simulink model "MPS_device_passive"  (R2018b)
settings: Solver=ode4  StartTime=0  StopTime=700  FixedStep=0.02  MaxStep=0.02  RelTol=1e-3  EnableMultiTasking=on
InitFcn:
  | %SSModel_calc
undefined symbols (not defined in the file): body, CentralPTOPreload, constraint, L, ML1Preload, ML2Preload, ML3Preload, ML4Preload, ML5Preload, ML6Preload, ML7Preload, ML8Preload, mrelative, pto, PTOrotation, SidePTO1Preload, SidePTO2Preload, SidePTO3Preload, SidePTO4Preload, simu, waves, X, Y, Z
libraries: nesl_utility x580, sm_lib x317, vrlib x72, WECSim_Lib x36
(part 24 of 27)

== system MPS_device_passive/PTO P2F2/VisuP2F3/Hydrodynamic Body/Morrison Element and ViscousDampingForceCalculation/Morrison Element Variant Subsystem/Morrison Element On/No Wave Morison Force/MorrisonElements/Rotation1 ==
  rot1 : Inport
  rot2 : Inport  Port=2
  rot3 : Inport  Port=3
  2 : Product
  3 : Product  Inputs=3
  7 : Product
  8 : Product  Inputs=3
  Combine : Concatenate  NumInputs=3  Mode=Multidimensional array  ConcatenateDimension=2
  Trigonometric Function{,1..2,6,9,11} (6 alike) : Trigonometry  Operator=cos
  Trigonometric Function{3..5,7..8,10} (6 alike) : Trigonometry
  rot11 : Product
  rot12 : Sum
  rot13 : Sum  Inputs=+-
  rot[1,1-3] : Outport
  wires:
  rot13/1 -> Combine/3
  8/1 -> rot13/2
  7/1 -> rot13/1
  Trigonometric Function11/1 -> 8/3
  Trigonometric Function10/1 -> 8/2
  Trigonometric Function9/1 -> 8/1
  Trigonometric Function8/1 -> 7/2
  Trigonometric Function7/1 -> 7/1
  rot1/1 -> Trigonometric Function7/1, Trigonometric Function9/1, Trigonometric Function4/1, Trigonometric Function2/1
  rot3/1 -> Trigonometric Function8/1, Trigonometric Function11/1, Trigonometric Function6/1, Trigonometric Function3/1, Trigonometric Function1/1
  rot2/1 -> Trigonometric Function10/1, Trigonometric Function5/1, Trigonometric Function/1
  Combine/1 -> rot[1,1-3]/1
  rot12/1 -> Combine/2
  3/1 -> rot12/2
  2/1 -> rot12/1
  Trigonometric Function6/1 -> 3/3
  Trigonometric Function5/1 -> 3/2
  Trigonometric Function4/1 -> 3/1
  Trigonometric Function3/1 -> 2/2
  Trigonometric Function2/1 -> 2/1
  rot11/1 -> Combine/1
  Trigonometric Function1/1 -> rot11/2
  Trigonometric Function/1 -> rot11/1

== system MPS_device_passive/PTO P2F2/VisuP2F3/Hydrodynamic Body/Morrison Element and ViscousDampingForceCalculation/Morrison Element Variant Subsystem/Morrison Element On/No Wave Morison Force/MorrisonElements/Rotation2 ==
  rot1 : Inport
  rot2 : Inport  Port=2
  rot3 : Inport  Port=3
  2 : Product
  3 : Product  Inputs=3
  7 : Product
  8 : Product  Inputs=3
  Combine : Concatenate  NumInputs=3  Mode=Multidimensional array  ConcatenateDimension=2
  Gain : Gain  Gain=-1
  Trigonometric Function{,2..3,8..9} (5 alike) : Trigonometry  Operator=cos
  Trigonometric Function{1,4..7,10..11} (7 alike) : Trigonometry
  rot11 : Product
  rot12 : Sum  Inputs=+-
  rot13 : Sum
  rot[2,1-3] : Outport
  wires:
  Gain/1 -> rot11/1
  rot13/1 -> Combine/3
  8/1 -> rot13/2
  7/1 -> rot13/1
  Trigonometric Function11/1 -> 8/3
  Trigonometric Function10/1 -> 8/2
  Trigonometric Function9/1 -> 8/1
  Trigonometric Function8/1 -> 7/2
  Trigonometric Function7/1 -> 7/1
  rot1/1 -> Trigonometric Function7/1, Trigonometric Function9/1, Trigonometric Function4/1, Trigonometric Function2/1
  rot3/1 -> Trigonometric Function8/1, Trigonometric Function11/1, Trigonometric Function6/1, Trigonometric Function3/1, Trigonometric Function1/1
  rot2/1 -> Trigonometric Function10/1, Trigonometric Function5/1, Trigonometric Function/1
  Combine/1 -> rot[2,1-3]/1
  rot12/1 -> Combine/2
  3/1 -> rot12/2
  2/1 -> rot12/1
  Trigonometric Function6/1 -> 3/3
  Trigonometric Function5/1 -> 3/2
  Trigonometric Function4/1 -> 3/1
  Trigonometric Function3/1 -> 2/2
  Trigonometric Function2/1 -> 2/1
  rot11/1 -> Combine/1
  Trigonometric Function1/1 -> rot11/2
  Trigonometric Function/1 -> Gain/1

== system MPS_device_passive/PTO P2F2/VisuP2F3/Hydrodynamic Body/Morrison Element and ViscousDampingForceCalculation/Morrison Element Variant Subsystem/Morrison Element On/No Wave Morison Force/MorrisonElements/Rotation3 ==
  rot1 : Inport
  rot2 : Inport  Port=2
  2 : Product
  7 : Product
  Combine : Concatenate  NumInputs=3  Mode=Multidimensional array  ConcatenateDimension=2
  Gain1 : Gain  Gain=-1
  TrigFun1 : Trigonometry
  TrigFun2 : Trigonometry
  TrigFun3 : Trigonometry  Operator=cos
  TrigFun4 : Trigonometry  Operator=cos
  TrigFun5 : Trigonometry  Operator=cos
  rot[3,1-3] : Outport
  wires:
  Gain1/1 -> 2/1
  TrigFun2/1 -> Gain1/1
  7/1 -> Combine/3
  rot1/1 -> TrigFun4/1, TrigFun2/1
  TrigFun5/1 -> 7/2
  TrigFun4/1 -> 7/1
  rot2/1 -> TrigFun1/1, TrigFun3/1, TrigFun5/1
  Combine/1 -> rot[3,1-3]/1
  2/1 -> Combine/2
  TrigFun3/1 -> 2/2
  TrigFun1/1 -> Combine/1

== system MPS_device_passive/PTO P2F2/VisuP2F3/Hydrodynamic Body/Morrison Element and ViscousDampingForceCalculation/Morrison Element Variant Subsystem/Morrison Element On/Regular Wave Morison Force/MorrisonElements/OrbitalVelocity ==
  Disp : Inport
  Time : Inport  Port=2
  MATLAB Function : MATLAB Function  TreatAsAtomicUnit=on
  WaveAmp : Constant  Value=waves.A(1,:)
  WaveFreq : Constant  Value=waves.w(1,:)
  WaveNumber : Constant  Value=waves.k(1,:)
  gravity : Constant  Value=simu.g  VectorParams1D=off
  phase : Constant  Value=0
  rampTime : Constant  Value=simu.rampT  VectorParams1D=off
  waterDepth : Constant  Value=waves.waterDepth  VectorParams1D=off
  waveDirection : Constant  Value=waves.waveDir  VectorParams1D=off
  u-V : Outport
  w-V : Outport  Port=2
  u-A : Outport  Port=3
  w-A : Outport  Port=4
  v-V : Outport  Port=5
  v-A : Outport  Port=6
  wires:
  MATLAB Function/5(ya) -> v-A/1
  MATLAB Function/1(u) -> u-V/1
  MATLAB Function/2(v) -> v-V/1
  MATLAB Function/6(za) -> w-A/1
  MATLAB Function/4(xa) -> u-A/1
  MATLAB Function/3(w) -> w-V/1
  rampTime/1 -> MATLAB Function/7(rampT)
  waveDirection/1 -> MATLAB Function/8(waveDir)
  waterDepth/1 -> MATLAB Function/9(waterDepth)
  gravity/1 -> MATLAB Function/10(g)
  Time/1 -> MATLAB Function/6(time)
  WaveAmp/1 -> MATLAB Function/4(waveAmp)
  WaveFreq/1 -> MATLAB Function/3(waveFreq)
  WaveNumber/1 -> MATLAB Function/2(waveNumber)
  phase/1 -> MATLAB Function/5(randPhase)
  Disp/1 -> MATLAB Function/1(disp)

== system MPS_device_passive/PTO P2F2/VisuP2F3/Hydrodynamic Body/Morrison Element and ViscousDampingForceCalculation/Morrison Element Variant Subsystem/Morrison Element On/Regular Wave Morison Force/MorrisonElements/Rotation1 ==
  rot1 : Inport
  rot2 : Inport  Port=2
  rot3 : Inport  Port=3
  2 : Product
  3 : Product  Inputs=3
  7 : Product
  8 : Product  Inputs=3
  Combine : Concatenate  NumInputs=3  Mode=Multidimensional array  ConcatenateDimension=2
  Trigonometric Function{,1..2,6,9,11} (6 alike) : Trigonometry  Operator=cos
  Trigonometric Function{3..5,7..8,10} (6 alike) : Trigonometry
  rot11 : Product
  rot12 : Sum
  rot13 : Sum  Inputs=+-
  rot[1,1-3] : Outport
  wires:
  rot13/1 -> Combine/3
  8/1 -> rot13/2
  7/1 -> rot13/1
  Trigonometric Function11/1 -> 8/3
  Trigonometric Function10/1 -> 8/2
  Trigonometric Function9/1 -> 8/1
  Trigonometric Function8/1 -> 7/2
  Trigonometric Function7/1 -> 7/1
  rot1/1 -> Trigonometric Function7/1, Trigonometric Function9/1, Trigonometric Function4/1, Trigonometric Function2/1
  rot3/1 -> Trigonometric Function8/1, Trigonometric Function11/1, Trigonometric Function6/1, Trigonometric Function3/1, Trigonometric Function1/1
  rot2/1 -> Trigonometric Function10/1, Trigonometric Function5/1, Trigonometric Function/1
  Combine/1 -> rot[1,1-3]/1
  rot12/1 -> Combine/2
  3/1 -> rot12/2
  2/1 -> rot12/1
  Trigonometric Function6/1 -> 3/3
  Trigonometric Function5/1 -> 3/2
  Trigonometric Function4/1 -> 3/1
  Trigonometric Function3/1 -> 2/2
  Trigonometric Function2/1 -> 2/1
  rot11/1 -> Combine/1
  Trigonometric Function1/1 -> rot11/2
  Trigonometric Function/1 -> rot11/1

== system MPS_device_passive/PTO P2F2/VisuP2F3/Hydrodynamic Body/Morrison Element and ViscousDampingForceCalculation/Morrison Element Variant Subsystem/Morrison Element On/Regular Wave Morison Force/MorrisonElements/Rotation2 ==
  rot1 : Inport
  rot2 : Inport  Port=2
  rot3 : Inport  Port=3
  2 : Product
  3 : Product  Inputs=3
  7 : Product
  8 : Product  Inputs=3
  Combine : Concatenate  NumInputs=3  Mode=Multidimensional array  ConcatenateDimension=2
  Gain : Gain  Gain=-1
  Trigonometric Function{,2..3,8..9} (5 alike) : Trigonometry  Operator=cos
  Trigonometric Function{1,4..7,10..11} (7 alike) : Trigonometry
  rot11 : Product
  rot12 : Sum  Inputs=+-
  rot13 : Sum
  rot[2,1-3] : Outport
  wires:
  Gain/1 -> rot11/1
  rot13/1 -> Combine/3
  8/1 -> rot13/2
  7/1 -> rot13/1
  Trigonometric Function11/1 -> 8/3
  Trigonometric Function10/1 -> 8/2
  Trigonometric Function9/1 -> 8/1
  Trigonometric Function8/1 -> 7/2
  Trigonometric Function7/1 -> 7/1
  rot1/1 -> Trigonometric Function7/1, Trigonometric Function9/1, Trigonometric Function4/1, Trigonometric Function2/1
  rot3/1 -> Trigonometric Function8/1, Trigonometric Function11/1, Trigonometric Function6/1, Trigonometric Function3/1, Trigonometric Function1/1
  rot2/1 -> Trigonometric Function10/1, Trigonometric Function5/1, Trigonometric Function/1
  Combine/1 -> rot[2,1-3]/1
  rot12/1 -> Combine/2
  3/1 -> rot12/2
  2/1 -> rot12/1
  Trigonometric Function6/1 -> 3/3
  Trigonometric Function5/1 -> 3/2
  Trigonometric Function4/1 -> 3/1
  Trigonometric Function3/1 -> 2/2
  Trigonometric Function2/1 -> 2/1
  rot11/1 -> Combine/1
  Trigonometric Function1/1 -> rot11/2
  Trigonometric Function/1 -> Gain/1

== system MPS_device_passive/PTO P2F2/VisuP2F3/Hydrodynamic Body/Morrison Element and ViscousDampingForceCalculation/Morrison Element Variant Subsystem/Morrison Element On/Regular Wave Morison Force/MorrisonElements/Rotation3 ==
  rot1 : Inport
  rot2 : Inport  Port=2
  2 : Product
  7 : Product
  Combine : Concatenate  NumInputs=3  Mode=Multidimensional array  ConcatenateDimension=2
  Gain1 : Gain  Gain=-1
  TrigFun1 : Trigonometry
  TrigFun2 : Trigonometry
  TrigFun3 : Trigonometry  Operator=cos
  TrigFun4 : Trigonometry  Operator=cos
  TrigFun5 : Trigonometry  Operator=cos
  rot[3,1-3] : Outport
  wires:
  Gain1/1 -> 2/1
  TrigFun2/1 -> Gain1/1
  7/1 -> Combine/3
  rot1/1 -> TrigFun4/1, TrigFun2/1
  TrigFun5/1 -> 7/2
  TrigFun4/1 -> 7/1
  rot2/1 -> TrigFun1/1, TrigFun3/1, TrigFun5/1
  Combine/1 -> rot[3,1-3]/1
  2/1 -> Combine/2
  TrigFun3/1 -> 2/2
  TrigFun1/1 -> Combine/1

== system MPS_device_passive/PTO P3F3/VisuP3F2/Hydrodynamic Body/Morrison Element and ViscousDampingForceCalculation/Morrison Element Variant Subsystem/Morrison Element On/Irregular Wave Morison Force/MorrisonElements/MorisonElementIrregular ==
  Disp : Inport
  waves.kirr : Inport  Port=2  Partition=on  PartitionDimension=1  PartitionWidth=1  PartitionOffset=0
  waves.w : Inport  Port=3  Partition=on  PartitionDimension=1  PartitionWidth=1  PartitionOffset=0
  waves.A : Inport  Port=4  Partition=on  PartitionDimension=1  PartitionWidth=1  PartitionOffset=0
  waves.RandPhase : Inport  Port=5  Partition=on  PartitionDimension=1  PartitionWidth=1  PartitionOffset=0
  Time : Inport  Port=6
  For Each : ForEach  DisableCoverage=on  IndexMode=One-based
  MATLAB Function : MATLAB Function  TreatAsAtomicUnit=on
  gravity : Constant  Value=simu.g  VectorParams1D=off
  rampTime : Constant  Value=simu.rampT  VectorParams1D=off
  waterDepth : Constant  Value=waves.waterDepth  VectorParams1D=off
  waveDirection : Constant  Value=waves.waveDir  VectorParams1D=off
  u-V : Outport  ConcatenationDimension=1
  w-V : Outport  Port=2  ConcatenationDimension=1
  x-A : Outport  Port=3  ConcatenationDimension=1
  w-A : Outport  Port=4  ConcatenationDimension=1
  v-V : Outport  Port=5  ConcatenationDimension=1
  y-A : Outport  Port=6  ConcatenationDimension=1
  wires:
  MATLAB Function/3(w) -> w-V/1
  MATLAB Function/4(xa) -> x-A/1
  MATLAB Function/6(za) -> w-A/1
  MATLAB Function/5(ya) -> y-A/1
  MATLAB Function/2(v) -> v-V/1
  Time/1 -> MATLAB Function/6(time)
  waves.kirr/1 -> MATLAB Function/2(waveNumber)
  MATLAB Function/1(u) -> u-V/1
  waves.RandPhase/1 -> MATLAB Function/5(randPhase)
  waves.A/1 -> MATLAB Function/4(waveAmp)
  waves.w/1 -> MATLAB Function/3(waveFreq)
  Disp/1 -> MATLAB Function/1(disp)
  rampTime/1 -> MATLAB Function/7(rampT)
  waveDirection/1 -> MATLAB Function/8(waveDir)
  waterDepth/1 -> MATLAB Function/9(waterDepth)
  gravity/1 -> MATLAB Function/10(g)

== system MPS_device_passive/PTO P3F3/VisuP3F2/Hydrodynamic Body/Morrison Element and ViscousDampingForceCalculation/Morrison Element Variant Subsystem/Morrison Element On/Irregular Wave Morison Force/MorrisonElements/Rotation1 ==
  rot1 : Inport
  rot2 : Inport  Port=2
  rot3 : Inport  Port=3
  2 : Product
  3 : Product  Inputs=3
  7 : Product
  8 : Product  Inputs=3
  Combine : Concatenate  NumInputs=3  Mode=Multidimensional array  ConcatenateDimension=2
  Trigonometric Function{,1..2,6,9,11} (6 alike) : Trigonometry  Operator=cos
  Trigonometric Function{3..5,7..8,10} (6 alike) : Trigonometry
  rot11 : Product
  rot12 : Sum
  rot13 : Sum  Inputs=+-
  rot[1,1-3] : Outport
  wires:
  rot13/1 -> Combine/3
  8/1 -> rot13/2
  7/1 -> rot13/1
  Trigonometric Function11/1 -> 8/3
  Trigonometric Function10/1 -> 8/2
  Trigonometric Function9/1 -> 8/1
  Trigonometric Function8/1 -> 7/2
  Trigonometric Function7/1 -> 7/1
  rot1/1 -> Trigonometric Function7/1, Trigonometric Function9/1, Trigonometric Function4/1, Trigonometric Function2/1
  rot3/1 -> Trigonometric Function8/1, Trigonometric Function11/1, Trigonometric Function6/1, Trigonometric Function3/1, Trigonometric Function1/1
  rot2/1 -> Trigonometric Function10/1, Trigonometric Function5/1, Trigonometric Function/1
  Combine/1 -> rot[1,1-3]/1
  rot12/1 -> Combine/2
  3/1 -> rot12/2
  2/1 -> rot12/1
  Trigonometric Function6/1 -> 3/3
  Trigonometric Function5/1 -> 3/2
  Trigonometric Function4/1 -> 3/1
  Trigonometric Function3/1 -> 2/2
  Trigonometric Function2/1 -> 2/1
  rot11/1 -> Combine/1
  Trigonometric Function1/1 -> rot11/2
  Trigonometric Function/1 -> rot11/1

== system MPS_device_passive/PTO P3F3/VisuP3F2/Hydrodynamic Body/Morrison Element and ViscousDampingForceCalculation/Morrison Element Variant Subsystem/Morrison Element On/Irregular Wave Morison Force/MorrisonElements/Rotation2 ==
  rot1 : Inport
  rot2 : Inport  Port=2
  rot3 : Inport  Port=3
  2 : Product
  3 : Product  Inputs=3
  7 : Product
  8 : Product  Inputs=3
  Combine : Concatenate  NumInputs=3  Mode=Multidimensional array  ConcatenateDimension=2
  Gain : Gain  Gain=-1
  Trigonometric Function{,2..3,8..9} (5 alike) : Trigonometry  Operator=cos
  Trigonometric Function{1,4..7,10..11} (7 alike) : Trigonometry
  rot11 : Product
  rot12 : Sum  Inputs=+-
  rot13 : Sum
  rot[2,1-3] : Outport
  wires:
  Gain/1 -> rot11/1
  rot13/1 -> Combine/3
  8/1 -> rot13/2
  7/1 -> rot13/1
  Trigonometric Function11/1 -> 8/3
  Trigonometric Function10/1 -> 8/2
  Trigonometric Function9/1 -> 8/1
  Trigonometric Function8/1 -> 7/2
  Trigonometric Function7/1 -> 7/1
  rot1/1 -> Trigonometric Function7/1, Trigonometric Function9/1, Trigonometric Function4/1, Trigonometric Function2/1
  rot3/1 -> Trigonometric Function8/1, Trigonometric Function11/1, Trigonometric Function6/1, Trigonometric Function3/1, Trigonometric Function1/1
  rot2/1 -> Trigonometric Function10/1, Trigonometric Function5/1, Trigonometric Function/1
  Combine/1 -> rot[2,1-3]/1
  rot12/1 -> Combine/2
  3/1 -> rot12/2
  2/1 -> rot12/1
  Trigonometric Function6/1 -> 3/3
  Trigonometric Function5/1 -> 3/2
  Trigonometric Function4/1 -> 3/1
  Trigonometric Function3/1 -> 2/2
  Trigonometric Function2/1 -> 2/1
  rot11/1 -> Combine/1
  Trigonometric Function1/1 -> rot11/2
  Trigonometric Function/1 -> Gain/1

== system MPS_device_passive/PTO P3F3/VisuP3F2/Hydrodynamic Body/Morrison Element and ViscousDampingForceCalculation/Morrison Element Variant Subsystem/Morrison Element On/Irregular Wave Morison Force/MorrisonElements/Rotation3 ==
  rot1 : Inport
  rot2 : Inport  Port=2
  2 : Product
  7 : Product
  Combine : Concatenate  NumInputs=3  Mode=Multidimensional array  ConcatenateDimension=2
  Gain1 : Gain  Gain=-1
  TrigFun1 : Trigonometry
  TrigFun2 : Trigonometry
  TrigFun3 : Trigonometry  Operator=cos
  TrigFun4 : Trigonometry  Operator=cos
  TrigFun5 : Trigonometry  Operator=cos
  rot[3,1-3] : Outport
  wires:
  Gain1/1 -> 2/1
  TrigFun2/1 -> Gain1/1
  7/1 -> Combine/3
  rot1/1 -> TrigFun4/1, TrigFun2/1
  TrigFun5/1 -> 7/2
  TrigFun4/1 -> 7/1
  rot2/1 -> TrigFun1/1, TrigFun3/1, TrigFun5/1
  Combine/1 -> rot[3,1-3]/1
  2/1 -> Combine/2
  TrigFun3/1 -> 2/2
  TrigFun1/1 -> Combine/1

== system MPS_device_passive/PTO P3F3/VisuP3F2/Hydrodynamic Body/Morrison Element and ViscousDampingForceCalculation/Morrison Element Variant Subsystem/Morrison Element On/No Wave Morison Force/MorrisonElements/OrbitalVelocity ==
  Disp : Inport
  Time : Inport  Port=2
  AmpMerge : Merge
  Applied Ramp Function : Subsystem  TreatAsAtomicUnit=on
  Disp-slx : Selector  InputPortWidth=3  IndexOptions=Index vector (dialog)  Indices=[1]  OutputSizes=1
  Disp-sly : Selector  InputPortWidth=3  IndexOptions=Index vector (dialog)  Indices=[2]  OutputSizes=1
  Disp-slz : Selector  InputPortWidth=3  IndexOptions=Index vector (dialog)  Indices=[3]  OutputSizes=1
  Gain : Gain  Gain=pi/180
  Gravity : Constant  Value=simu.g
  HorizHead : Trigonometry  Operator=cos
  Horizontal-x,y : Trigonometry  Operator=cos
  Horizontal-z : Trigonometry  Operator=cosh
  No Ramp Function : Subsystem  TreatAsAtomicUnit=on
  Ramp : If  NumInputs=2  IfExpression=u1 < u2
  Ramp Function Time : Constant  Value=simu.rampT
  VertHead : Trigonometry
  Vertical-x,y : Trigonometry
  Vertical-z : Trigonometry  Operator=sinh
  WaterDepth : Constant  Value=waves.waterDepth
  WaveAmp : Constant  Value=waves.A(1,:)
  WaveFreq : Constant  Value=waves.w(1,:)
  WaveHeading : Constant  Value=waves.waveDir
  WaveNumber : Constant  Value=waves.k(1,:)
  X-A : Gain  Gain=-1
  Y-A : Gain  Gain=-1
  Y-V : Gain  Gain=-1
  Z-A : Gain  Gain=-1
  cosh : Trigonometry  Operator=cosh
  cosh*cos : Product  Inputs=**
  cosh*sin : Product  Inputs=**
  cosh/coshkh : Product  Inputs=*/
  k(xcos + ysin) : Sum
  k*h : Product
  k*x*cos(beta) : Product  Inputs=3
  k*y*sin(beta) : Product  Inputs=3
  k*z : Product
  sigma*t : Product
  sincos : Sum  Inputs=-+
  sinh*cos : Product  Inputs=**
  sinh*sin : Product  Inputs=**
  sinh/coshkh : Product  Inputs=*/
  sinhcosh : Sum
  u-Accel : Product  Inputs=*****
  u-Vel : Product  Inputs=****/*
  u-Vel1 : Product  Inputs=****/*
  v-Accel : Product  Inputs=*****
  w-Accel : Product  Inputs=****
  w-Vel : Product  Inputs=****/
  u-V : Outport
  w-V : Outport  Port=2
  u-A : Outport  Port=3
  w-A : Outport  Port=4
  v-V : Outport  Port=5
  v-A : Outport  Port=6
  wires:
  v-Accel/1 -> v-A/1
  Y-A/1 -> v-Accel/1
  u-Vel/1 -> u-V/1
  u-Vel1/1 -> v-V/1
  k(xcos + ysin)/1 -> sincos/1
  k*x*cos(beta)/1 -> k(xcos + ysin)/1
  k*y*sin(beta)/1 -> k(xcos + ysin)/2
  VertHead/1 -> v-Accel/5, u-Vel1/6, k*y*sin(beta)/1
  HorizHead/1 -> k*x*cos(beta)/1, u-Vel/6, u-Accel/5
  Disp-slx/1 -> k*x*cos(beta)/2
  Gain/1 -> VertHead/1, HorizHead/1
  WaveHeading/1 -> Gain/1
  WaveAmp/1 -> No Ramp Function/1(Ain), Applied Ramp Function/1(Ain)
  WaveFreq/1 -> sigma*t/1, u-Vel/5, u-Vel1/5, w-Vel/5
  Disp-slz/1 -> k*z/1
  Applied Ramp Function/1(Aout) -> AmpMerge/1
  No Ramp Function/1(Aout) -> AmpMerge/2
  Time/1 -> sigma*t/2, Ramp/1
  Ramp/1 -> Applied Ramp Function/Action
  Ramp/2 -> No Ramp Function/Action
  Ramp Function Time/1 -> Ramp/2
  sinh*cos/1 -> Z-A/1
  cosh*sin/1 -> X-A/1, Y-A/1
  w-Accel/1 -> w-A/1
  u-Accel/1 -> u-A/1
  w-Vel/1 -> w-V/1
  Z-A/1 -> w-Accel/1
  X-A/1 -> u-Accel/1
  Y-V/1 -> w-Vel/1
  sinh*sin/1 -> Y-V/1
  Gravity/1 -> u-Vel/3, u-Vel1/3, u-Accel/3, w-Accel/3, v-Accel/3, w-Vel/3
  AmpMerge/1 -> u-Vel/2, u-Vel1/2, u-Accel/2, v-Accel/2, w-Accel/2, w-Vel/2
  cosh*cos/1 -> u-Vel/1, u-Vel1/1
  Disp-sly/1 -> k*y*sin(beta)/2
  cosh/coshkh/1 -> cosh*sin/2, cosh*cos/2
  Horizontal-x,y/1 -> cosh*cos/1, sinh*cos/1
  sinh/coshkh/1 -> sinh*sin/2, sinh*cos/2
  Vertical-x,y/1 -> sinh*sin/1, cosh*sin/1
  Vertical-z/1 -> sinh/coshkh/1
  cosh/1 -> cosh/coshkh/2, sinh/coshkh/2
  Horizontal-z/1 -> cosh/coshkh/1
  sinhcosh/1 -> Horizontal-z/1, Vertical-z/1
  k*h/1 -> sinhcosh/2, cosh/1
  k*z/1 -> sinhcosh/1
  sincos/1 -> Horizontal-x,y/1, Vertical-x,y/1
  sigma*t/1 -> sincos/2
  WaterDepth/1 -> k*h/1
  WaveNumber/1 -> u-Vel/4, u-Vel1/4, u-Accel/4, w-Accel/4, v-Accel/4, w-Vel/4, k*x*cos(beta)/3, k*y*sin(beta)/3, k*z/2, k*h/2
  Disp/1 -> Disp-slx/1, Disp-sly/1, Disp-slz/1

== system MPS_device_passive/PTO P3F3/VisuP3F2/Hydrodynamic Body/Morrison Element and ViscousDampingForceCalculation/Morrison Element Variant Subsystem/Morrison Element On/No Wave Morison Force/MorrisonElements/Rotation1 ==
  rot1 : Inport
  rot2 : Inport  Port=2
  rot3 : Inport  Port=3
  2 : Product
  3 : Product  Inputs=3
  7 : Product
  8 : Product  Inputs=3
  Combine : Concatenate  NumInputs=3  Mode=Multidimensional array  ConcatenateDimension=2
  Trigonometric Function{,1..2,6,9,11} (6 alike) : Trigonometry  Operator=cos
  Trigonometric Function{3..5,7..8,10} (6 alike) : Trigonometry
  rot11 : Product
  rot12 : Sum
  rot13 : Sum  Inputs=+-
  rot[1,1-3] : Outport
  wires:
  rot13/1 -> Combine/3
  8/1 -> rot13/2
  7/1 -> rot13/1
  Trigonometric Function11/1 -> 8/3
  Trigonometric Function10/1 -> 8/2
  Trigonometric Function9/1 -> 8/1
  Trigonometric Function8/1 -> 7/2
  Trigonometric Function7/1 -> 7/1
  rot1/1 -> Trigonometric Function7/1, Trigonometric Function9/1, Trigonometric Function4/1, Trigonometric Function2/1
  rot3/1 -> Trigonometric Function8/1, Trigonometric Function11/1, Trigonometric Function6/1, Trigonometric Function3/1, Trigonometric Function1/1
  rot2/1 -> Trigonometric Function10/1, Trigonometric Function5/1, Trigonometric Function/1
  Combine/1 -> rot[1,1-3]/1
  rot12/1 -> Combine/2
  3/1 -> rot12/2
  2/1 -> rot12/1
  Trigonometric Function6/1 -> 3/3
  Trigonometric Function5/1 -> 3/2
  Trigonometric Function4/1 -> 3/1
  Trigonometric Function3/1 -> 2/2
  Trigonometric Function2/1 -> 2/1
  rot11/1 -> Combine/1
  Trigonometric Function1/1 -> rot11/2
  Trigonometric Function/1 -> rot11/1

== system MPS_device_passive/PTO P3F3/VisuP3F2/Hydrodynamic Body/Morrison Element and ViscousDampingForceCalculation/Morrison Element Variant Subsystem/Morrison Element On/No Wave Morison Force/MorrisonElements/Rotation2 ==
  rot1 : Inport
  rot2 : Inport  Port=2
  rot3 : Inport  Port=3
  2 : Product
  3 : Product  Inputs=3
  7 : Product
  8 : Product  Inputs=3
  Combine : Concatenate  NumInputs=3  Mode=Multidimensional array  ConcatenateDimension=2
  Gain : Gain  Gain=-1
  Trigonometric Function{,2..3,8..9} (5 alike) : Trigonometry  Operator=cos
  Trigonometric Function{1,4..7,10..11} (7 alike) : Trigonometry
  rot11 : Product
  rot12 : Sum  Inputs=+-
  rot13 : Sum
  rot[2,1-3] : Outport
  wires:
  Gain/1 -> rot11/1
  rot13/1 -> Combine/3
  8/1 -> rot13/2
  7/1 -> rot13/1
  Trigonometric Function11/1 -> 8/3
  Trigonometric Function10/1 -> 8/2
  Trigonometric Function9/1 -> 8/1
  Trigonometric Function8/1 -> 7/2
  Trigonometric Function7/1 -> 7/1
  rot1/1 -> Trigonometric Function7/1, Trigonometric Function9/1, Trigonometric Function4/1, Trigonometric Function2/1
  rot3/1 -> Trigonometric Function8/1, Trigonometric Function11/1, Trigonometric Function6/1, Trigonometric Function3/1, Trigonometric Function1/1
  rot2/1 -> Trigonometric Function10/1, Trigonometric Function5/1, Trigonometric Function/1
  Combine/1 -> rot[2,1-3]/1
  rot12/1 -> Combine/2
  3/1 -> rot12/2
  2/1 -> rot12/1
  Trigonometric Function6/1 -> 3/3
  Trigonometric Function5/1 -> 3/2
  Trigonometric Function4/1 -> 3/1
  Trigonometric Function3/1 -> 2/2
  Trigonometric Function2/1 -> 2/1
  rot11/1 -> Combine/1
  Trigonometric Function1/1 -> rot11/2
  Trigonometric Function/1 -> Gain/1

== system MPS_device_passive/PTO P3F3/VisuP3F2/Hydrodynamic Body/Morrison Element and ViscousDampingForceCalculation/Morrison Element Variant Subsystem/Morrison Element On/No Wave Morison Force/MorrisonElements/Rotation3 ==
  rot1 : Inport
  rot2 : Inport  Port=2
  2 : Product
  7 : Product
  Combine : Concatenate  NumInputs=3  Mode=Multidimensional array  ConcatenateDimension=2
  Gain1 : Gain  Gain=-1
  TrigFun1 : Trigonometry
  TrigFun2 : Trigonometry
  TrigFun3 : Trigonometry  Operator=cos
  TrigFun4 : Trigonometry  Operator=cos
  TrigFun5 : Trigonometry  Operator=cos
  rot[3,1-3] : Outport
  wires:
  Gain1/1 -> 2/1
  TrigFun2/1 -> Gain1/1
  7/1 -> Combine/3
  rot1/1 -> TrigFun4/1, TrigFun2/1
  TrigFun5/1 -> 7/2
  TrigFun4/1 -> 7/1
  rot2/1 -> TrigFun1/1, TrigFun3/1, TrigFun5/1
  Combine/1 -> rot[3,1-3]/1
  2/1 -> Combine/2
  TrigFun3/1 -> 2/2
  TrigFun1/1 -> Combine/1

== system MPS_device_passive/PTO P3F3/VisuP3F2/Hydrodynamic Body/Morrison Element and ViscousDampingForceCalculation/Morrison Element Variant Subsystem/Morrison Element On/Regular Wave Morison Force/MorrisonElements/OrbitalVelocity ==
  Disp : Inport
  Time : Inport  Port=2
  MATLAB Function : MATLAB Function  TreatAsAtomicUnit=on
  WaveAmp : Constant  Value=waves.A(1,:)
  WaveFreq : Constant  Value=waves.w(1,:)
  WaveNumber : Constant  Value=waves.k(1,:)
  gravity : Constant  Value=simu.g  VectorParams1D=off
  phase : Constant  Value=0
  rampTime : Constant  Value=simu.rampT  VectorParams1D=off
  waterDepth : Constant  Value=waves.waterDepth  VectorParams1D=off
  waveDirection : Constant  Value=waves.waveDir  VectorParams1D=off
  u-V : Outport
  w-V : Outport  Port=2
  u-A : Outport  Port=3
  w-A : Outport  Port=4
  v-V : Outport  Port=5
  v-A : Outport  Port=6
  wires:
  MATLAB Function/5(ya) -> v-A/1
  MATLAB Function/1(u) -> u-V/1
  MATLAB Function/2(v) -> v-V/1
  MATLAB Function/6(za) -> w-A/1
  MATLAB Function/4(xa) -> u-A/1
  MATLAB Function/3(w) -> w-V/1
  rampTime/1 -> MATLAB Function/7(rampT)
  waveDirection/1 -> MATLAB Function/8(waveDir)
  waterDepth/1 -> MATLAB Function/9(waterDepth)
  gravity/1 -> MATLAB Function/10(g)
  Time/1 -> MATLAB Function/6(time)
  WaveAmp/1 -> MATLAB Function/4(waveAmp)
  WaveFreq/1 -> MATLAB Function/3(waveFreq)
  WaveNumber/1 -> MATLAB Function/2(waveNumber)
  phase/1 -> MATLAB Function/5(randPhase)
  Disp/1 -> MATLAB Function/1(disp)

== system MPS_device_passive/PTO P3F3/VisuP3F2/Hydrodynamic Body/Morrison Element and ViscousDampingForceCalculation/Morrison Element Variant Subsystem/Morrison Element On/Regular Wave Morison Force/MorrisonElements/Rotation1 ==
  rot1 : Inport
  rot2 : Inport  Port=2
  rot3 : Inport  Port=3
  2 : Product
  3 : Product  Inputs=3
  7 : Product
  8 : Product  Inputs=3
  Combine : Concatenate  NumInputs=3  Mode=Multidimensional array  ConcatenateDimension=2
  Trigonometric Function{,1..2,6,9,11} (6 alike) : Trigonometry  Operator=cos
  Trigonometric Function{3..5,7..8,10} (6 alike) : Trigonometry
  rot11 : Product
  rot12 : Sum
  rot13 : Sum  Inputs=+-
  rot[1,1-3] : Outport
  wires:
  rot13/1 -> Combine/3
  8/1 -> rot13/2
  7/1 -> rot13/1
  Trigonometric Function11/1 -> 8/3
  Trigonometric Function10/1 -> 8/2
  Trigonometric Function9/1 -> 8/1
  Trigonometric Function8/1 -> 7/2
  Trigonometric Function7/1 -> 7/1
  rot1/1 -> Trigonometric Function7/1, Trigonometric Function9/1, Trigonometric Function4/1, Trigonometric Function2/1
  rot3/1 -> Trigonometric Function8/1, Trigonometric Function11/1, Trigonometric Function6/1, Trigonometric Function3/1, Trigonometric Function1/1
  rot2/1 -> Trigonometric Function10/1, Trigonometric Function5/1, Trigonometric Function/1
  Combine/1 -> rot[1,1-3]/1
  rot12/1 -> Combine/2
  3/1 -> rot12/2
  2/1 -> rot12/1
  Trigonometric Function6/1 -> 3/3
  Trigonometric Function5/1 -> 3/2
  Trigonometric Function4/1 -> 3/1
  Trigonometric Function3/1 -> 2/2
  Trigonometric Function2/1 -> 2/1
  rot11/1 -> Combine/1
  Trigonometric Function1/1 -> rot11/2
  Trigonometric Function/1 -> rot11/1

== system MPS_device_passive/PTO P3F3/VisuP3F2/Hydrodynamic Body/Morrison Element and ViscousDampingForceCalculation/Morrison Element Variant Subsystem/Morrison Element On/Regular Wave Morison Force/MorrisonElements/Rotation2 ==
  rot1 : Inport
  rot2 : Inport  Port=2
  rot3 : Inport  Port=3
  2 : Product
  3 : Product  Inputs=3
  7 : Product
  8 : Product  Inputs=3
  Combine : Concatenate  NumInputs=3  Mode=Multidimensional array  ConcatenateDimension=2
  Gain : Gain  Gain=-1
  Trigonometric Function{,2..3,8..9} (5 alike) : Trigonometry  Operator=cos
  Trigonometric Function{1,4..7,10..11} (7 alike) : Trigonometry
  rot11 : Product
  rot12 : Sum  Inputs=+-
  rot13 : Sum
  rot[2,1-3] : Outport
  wires:
  Gain/1 -> rot11/1
  rot13/1 -> Combine/3
  8/1 -> rot13/2
  7/1 -> rot13/1
  Trigonometric Function11/1 -> 8/3
  Trigonometric Function10/1 -> 8/2
  Trigonometric Function9/1 -> 8/1
  Trigonometric Function8/1 -> 7/2
  Trigonometric Function7/1 -> 7/1
  rot1/1 -> Trigonometric Function7/1, Trigonometric Function9/1, Trigonometric Function4/1, Trigonometric Function2/1
  rot3/1 -> Trigonometric Function8/1, Trigonometric Function11/1, Trigonometric Function6/1, Trigonometric Function3/1, Trigonometric Function1/1
  rot2/1 -> Trigonometric Function10/1, Trigonometric Function5/1, Trigonometric Function/1
  Combine/1 -> rot[2,1-3]/1
  rot12/1 -> Combine/2
  3/1 -> rot12/2
  2/1 -> rot12/1
  Trigonometric Function6/1 -> 3/3
  Trigonometric Function5/1 -> 3/2
  Trigonometric Function4/1 -> 3/1
  Trigonometric Function3/1 -> 2/2
  Trigonometric Function2/1 -> 2/1
  rot11/1 -> Combine/1
  Trigonometric Function1/1 -> rot11/2
  Trigonometric Function/1 -> Gain/1

== system MPS_device_passive/PTO P3F3/VisuP3F2/Hydrodynamic Body/Morrison Element and ViscousDampingForceCalculation/Morrison Element Variant Subsystem/Morrison Element On/Regular Wave Morison Force/MorrisonElements/Rotation3 ==
  rot1 : Inport
  rot2 : Inport  Port=2
  2 : Product
  7 : Product
  Combine : Concatenate  NumInputs=3  Mode=Multidimensional array  ConcatenateDimension=2
  Gain1 : Gain  Gain=-1
  TrigFun1 : Trigonometry
  TrigFun2 : Trigonometry
  TrigFun3 : Trigonometry  Operator=cos
  TrigFun4 : Trigonometry  Operator=cos
  TrigFun5 : Trigonometry  Operator=cos
  rot[3,1-3] : Outport
  wires:
  Gain1/1 -> 2/1
  TrigFun2/1 -> Gain1/1
  7/1 -> Combine/3
  rot1/1 -> TrigFun4/1, TrigFun2/1
  TrigFun5/1 -> 7/2
  TrigFun4/1 -> 7/1
  rot2/1 -> TrigFun1/1, TrigFun3/1, TrigFun5/1
  Combine/1 -> rot[3,1-3]/1
  2/1 -> Combine/2
  TrigFun3/1 -> 2/2
  TrigFun1/1 -> Combine/1

== system MPS_device_passive/PTO P4F4/VisuP4F1/Hydrodynamic Body/Morrison Element and ViscousDampingForceCalculation/Morrison Element Variant Subsystem/Morrison Element On/Irregular Wave Morison Force/MorrisonElements/MorisonElementIrregular ==
  Disp : Inport
  waves.kirr : Inport  Port=2  Partition=on  PartitionDimension=1  PartitionWidth=1  PartitionOffset=0
  waves.w : Inport  Port=3  Partition=on  PartitionDimension=1  PartitionWidth=1  PartitionOffset=0
  waves.A : Inport  Port=4  Partition=on  PartitionDimension=1  PartitionWidth=1  PartitionOffset=0
  waves.RandPhase : Inport  Port=5  Partition=on  PartitionDimension=1  PartitionWidth=1  PartitionOffset=0
  Time : Inport  Port=6
  For Each : ForEach  DisableCoverage=on  IndexMode=One-based
  MATLAB Function : MATLAB Function  TreatAsAtomicUnit=on
  gravity : Constant  Value=simu.g  VectorParams1D=off
  rampTime : Constant  Value=simu.rampT  VectorParams1D=off
  waterDepth : Constant  Value=waves.waterDepth  VectorParams1D=off
  waveDirection : Constant  Value=waves.waveDir  VectorParams1D=off
  u-V : Outport  ConcatenationDimension=1
  w-V : Outport  Port=2  ConcatenationDimension=1
  x-A : Outport  Port=3  ConcatenationDimension=1
  w-A : Outport  Port=4  ConcatenationDimension=1
  v-V : Outport  Port=5  ConcatenationDimension=1
  y-A : Outport  Port=6  ConcatenationDimension=1
  wires:
  MATLAB Function/3(w) -> w-V/1
  MATLAB Function/4(xa) -> x-A/1
  MATLAB Function/6(za) -> w-A/1
  MATLAB Function/5(ya) -> y-A/1
  MATLAB Function/2(v) -> v-V/1
  Time/1 -> MATLAB Function/6(time)
  waves.kirr/1 -> MATLAB Function/2(waveNumber)
  MATLAB Function/1(u) -> u-V/1
  waves.RandPhase/1 -> MATLAB Function/5(randPhase)
  waves.A/1 -> MATLAB Function/4(waveAmp)
  waves.w/1 -> MATLAB Function/3(waveFreq)
  Disp/1 -> MATLAB Function/1(disp)
  rampTime/1 -> MATLAB Function/7(rampT)
  waveDirection/1 -> MATLAB Function/8(waveDir)
  waterDepth/1 -> MATLAB Function/9(waterDepth)
  gravity/1 -> MATLAB Function/10(g)

== system MPS_device_passive/PTO P4F4/VisuP4F1/Hydrodynamic Body/Morrison Element and ViscousDampingForceCalculation/Morrison Element Variant Subsystem/Morrison Element On/Irregular Wave Morison Force/MorrisonElements/Rotation1 ==
  rot1 : Inport
  rot2 : Inport  Port=2
  rot3 : Inport  Port=3
  2 : Product
  3 : Product  Inputs=3
  7 : Product
  8 : Product  Inputs=3
  Combine : Concatenate  NumInputs=3  Mode=Multidimensional array  ConcatenateDimension=2
  Trigonometric Function{,1..2,6,9,11} (6 alike) : Trigonometry  Operator=cos
  Trigonometric Function{3..5,7..8,10} (6 alike) : Trigonometry
  rot11 : Product
  rot12 : Sum
  rot13 : Sum  Inputs=+-
  rot[1,1-3] : Outport
  wires:
  rot13/1 -> Combine/3
  8/1 -> rot13/2
  7/1 -> rot13/1
  Trigonometric Function11/1 -> 8/3
  Trigonometric Function10/1 -> 8/2
  Trigonometric Function9/1 -> 8/1
  Trigonometric Function8/1 -> 7/2
  Trigonometric Function7/1 -> 7/1
  rot1/1 -> Trigonometric Function7/1, Trigonometric Function9/1, Trigonometric Function4/1, Trigonometric Function2/1
  rot3/1 -> Trigonometric Function8/1, Trigonometric Function11/1, Trigonometric Function6/1, Trigonometric Function3/1, Trigonometric Function1/1
  rot2/1 -> Trigonometric Function10/1, Trigonometric Function5/1, Trigonometric Function/1
  Combine/1 -> rot[1,1-3]/1
  rot12/1 -> Combine/2
  3/1 -> rot12/2
  2/1 -> rot12/1
  Trigonometric Function6/1 -> 3/3
  Trigonometric Function5/1 -> 3/2
  Trigonometric Function4/1 -> 3/1
  Trigonometric Function3/1 -> 2/2
  Trigonometric Function2/1 -> 2/1
  rot11/1 -> Combine/1
  Trigonometric Function1/1 -> rot11/2
  Trigonometric Function/1 -> rot11/1

== system MPS_device_passive/PTO P4F4/VisuP4F1/Hydrodynamic Body/Morrison Element and ViscousDampingForceCalculation/Morrison Element Variant Subsystem/Morrison Element On/Irregular Wave Morison Force/MorrisonElements/Rotation2 ==
  rot1 : Inport
  rot2 : Inport  Port=2
  rot3 : Inport  Port=3
  2 : Product
  3 : Product  Inputs=3
  7 : Product
  8 : Product  Inputs=3
  Combine : Concatenate  NumInputs=3  Mode=Multidimensional array  ConcatenateDimension=2
  Gain : Gain  Gain=-1
  Trigonometric Function{,2..3,8..9} (5 alike) : Trigonometry  Operator=cos
  Trigonometric Function{1,4..7,10..11} (7 alike) : Trigonometry
  rot11 : Product
  rot12 : Sum  Inputs=+-
  rot13 : Sum
  rot[2,1-3] : Outport
  wires:
  Gain/1 -> rot11/1
  rot13/1 -> Combine/3
  8/1 -> rot13/2
  7/1 -> rot13/1
  Trigonometric Function11/1 -> 8/3
  Trigonometric Function10/1 -> 8/2
  Trigonometric Function9/1 -> 8/1
  Trigonometric Function8/1 -> 7/2
  Trigonometric Function7/1 -> 7/1
  rot1/1 -> Trigonometric Function7/1, Trigonometric Function9/1, Trigonometric Function4/1, Trigonometric Function2/1
  rot3/1 -> Trigonometric Function8/1, Trigonometric Function11/1, Trigonometric Function6/1, Trigonometric Function3/1, Trigonometric Function1/1
  rot2/1 -> Trigonometric Function10/1, Trigonometric Function5/1, Trigonometric Function/1
  Combine/1 -> rot[2,1-3]/1
  rot12/1 -> Combine/2
  3/1 -> rot12/2
  2/1 -> rot12/1
  Trigonometric Function6/1 -> 3/3
  Trigonometric Function5/1 -> 3/2
  Trigonometric Function4/1 -> 3/1
  Trigonometric Function3/1 -> 2/2
  Trigonometric Function2/1 -> 2/1
  rot11/1 -> Combine/1
  Trigonometric Function1/1 -> rot11/2
  Trigonometric Function/1 -> Gain/1

== system MPS_device_passive/PTO P4F4/VisuP4F1/Hydrodynamic Body/Morrison Element and ViscousDampingForceCalculation/Morrison Element Variant Subsystem/Morrison Element On/Irregular Wave Morison Force/MorrisonElements/Rotation3 ==
  rot1 : Inport
  rot2 : Inport  Port=2
  2 : Product
  7 : Product
  Combine : Concatenate  NumInputs=3  Mode=Multidimensional array  ConcatenateDimension=2
  Gain1 : Gain  Gain=-1
  TrigFun1 : Trigonometry
  TrigFun2 : Trigonometry
  TrigFun3 : Trigonometry  Operator=cos
  TrigFun4 : Trigonometry  Operator=cos
  TrigFun5 : Trigonometry  Operator=cos
  rot[3,1-3] : Outport
  wires:
  Gain1/1 -> 2/1
  TrigFun2/1 -> Gain1/1
  7/1 -> Combine/3
  rot1/1 -> TrigFun4/1, TrigFun2/1
  TrigFun5/1 -> 7/2
  TrigFun4/1 -> 7/1
  rot2/1 -> TrigFun1/1, TrigFun3/1, TrigFun5/1
  Combine/1 -> rot[3,1-3]/1
  2/1 -> Combine/2
  TrigFun3/1 -> 2/2
  TrigFun1/1 -> Combine/1

== system MPS_device_passive/PTO P4F4/VisuP4F1/Hydrodynamic Body/Morrison Element and ViscousDampingForceCalculation/Morrison Element Variant Subsystem/Morrison Element On/No Wave Morison Force/MorrisonElements/OrbitalVelocity ==
  Disp : Inport
  Time : Inport  Port=2
  AmpMerge : Merge
  Applied Ramp Function : Subsystem  TreatAsAtomicUnit=on
  Disp-slx : Selector  InputPortWidth=3  IndexOptions=Index vector (dialog)  Indices=[1]  OutputSizes=1
  Disp-sly : Selector  InputPortWidth=3  IndexOptions=Index vector (dialog)  Indices=[2]  OutputSizes=1
  Disp-slz : Selector  InputPortWidth=3  IndexOptions=Index vector (dialog)  Indices=[3]  OutputSizes=1
  Gain : Gain  Gain=pi/180
  Gravity : Constant  Value=simu.g
  HorizHead : Trigonometry  Operator=cos
  Horizontal-x,y : Trigonometry  Operator=cos
  Horizontal-z : Trigonometry  Operator=cosh
  No Ramp Function : Subsystem  TreatAsAtomicUnit=on
  Ramp : If  NumInputs=2  IfExpression=u1 < u2
  Ramp Function Time : Constant  Value=simu.rampT
  VertHead : Trigonometry
  Vertical-x,y : Trigonometry
  Vertical-z : Trigonometry  Operator=sinh
  WaterDepth : Constant  Value=waves.waterDepth
  WaveAmp : Constant  Value=waves.A(1,:)
  WaveFreq : Constant  Value=waves.w(1,:)
  WaveHeading : Constant  Value=waves.waveDir
  WaveNumber : Constant  Value=waves.k(1,:)
  X-A : Gain  Gain=-1
  Y-A : Gain  Gain=-1
  Y-V : Gain  Gain=-1
  Z-A : Gain  Gain=-1
  cosh : Trigonometry  Operator=cosh
  cosh*cos : Product  Inputs=**
  cosh*sin : Product  Inputs=**
  cosh/coshkh : Product  Inputs=*/
  k(xcos + ysin) : Sum
  k*h : Product
  k*x*cos(beta) : Product  Inputs=3
  k*y*sin(beta) : Product  Inputs=3
  k*z : Product
  sigma*t : Product
  sincos : Sum  Inputs=-+
  sinh*cos : Product  Inputs=**
  sinh*sin : Product  Inputs=**
  sinh/coshkh : Product  Inputs=*/
  sinhcosh : Sum
  u-Accel : Product  Inputs=*****
  u-Vel : Product  Inputs=****/*
  u-Vel1 : Product  Inputs=****/*
  v-Accel : Product  Inputs=*****
  w-Accel : Product  Inputs=****
  w-Vel : Product  Inputs=****/
  u-V : Outport
  w-V : Outport  Port=2
  u-A : Outport  Port=3
  w-A : Outport  Port=4
  v-V : Outport  Port=5
  v-A : Outport  Port=6
  wires:
  v-Accel/1 -> v-A/1
  Y-A/1 -> v-Accel/1
  u-Vel/1 -> u-V/1
  u-Vel1/1 -> v-V/1
  k(xcos + ysin)/1 -> sincos/1
  k*x*cos(beta)/1 -> k(xcos + ysin)/1
  k*y*sin(beta)/1 -> k(xcos + ysin)/2
  VertHead/1 -> v-Accel/5, u-Vel1/6, k*y*sin(beta)/1
  HorizHead/1 -> k*x*cos(beta)/1, u-Vel/6, u-Accel/5
  Disp-slx/1 -> k*x*cos(beta)/2
  Gain/1 -> VertHead/1, HorizHead/1
  WaveHeading/1 -> Gain/1
  WaveAmp/1 -> No Ramp Function/1(Ain), Applied Ramp Function/1(Ain)
  WaveFreq/1 -> sigma*t/1, u-Vel/5, u-Vel1/5, w-Vel/5
  Disp-slz/1 -> k*z/1
  Applied Ramp Function/1(Aout) -> AmpMerge/1
  No Ramp Function/1(Aout) -> AmpMerge/2
  Time/1 -> sigma*t/2, Ramp/1
  Ramp/1 -> Applied Ramp Function/Action
  Ramp/2 -> No Ramp Function/Action
  Ramp Function Time/1 -> Ramp/2
  sinh*cos/1 -> Z-A/1
  cosh*sin/1 -> X-A/1, Y-A/1
  w-Accel/1 -> w-A/1
  u-Accel/1 -> u-A/1
  w-Vel/1 -> w-V/1
  Z-A/1 -> w-Accel/1
  X-A/1 -> u-Accel/1
  Y-V/1 -> w-Vel/1
  sinh*sin/1 -> Y-V/1
  Gravity/1 -> u-Vel/3, u-Vel1/3, u-Accel/3, w-Accel/3, v-Accel/3, w-Vel/3
  AmpMerge/1 -> u-Vel/2, u-Vel1/2, u-Accel/2, v-Accel/2, w-Accel/2, w-Vel/2
  cosh*cos/1 -> u-Vel/1, u-Vel1/1
  Disp-sly/1 -> k*y*sin(beta)/2
  cosh/coshkh/1 -> cosh*sin/2, cosh*cos/2
  Horizontal-x,y/1 -> cosh*cos/1, sinh*cos/1
  sinh/coshkh/1 -> sinh*sin/2, sinh*cos/2
  Vertical-x,y/1 -> sinh*sin/1, cosh*sin/1
  Vertical-z/1 -> sinh/coshkh/1
  cosh/1 -> cosh/coshkh/2, sinh/coshkh/2
  Horizontal-z/1 -> cosh/coshkh/1
  sinhcosh/1 -> Horizontal-z/1, Vertical-z/1
  k*h/1 -> sinhcosh/2, cosh/1
  k*z/1 -> sinhcosh/1
  sincos/1 -> Horizontal-x,y/1, Vertical-x,y/1
  sigma*t/1 -> sincos/2
  WaterDepth/1 -> k*h/1
  WaveNumber/1 -> u-Vel/4, u-Vel1/4, u-Accel/4, w-Accel/4, v-Accel/4, w-Vel/4, k*x*cos(beta)/3, k*y*sin(beta)/3, k*z/2, k*h/2
  Disp/1 -> Disp-slx/1, Disp-sly/1, Disp-slz/1

== system MPS_device_passive/PTO P4F4/VisuP4F1/Hydrodynamic Body/Morrison Element and ViscousDampingForceCalculation/Morrison Element Variant Subsystem/Morrison Element On/No Wave Morison Force/MorrisonElements/Rotation1 ==
  rot1 : Inport
  rot2 : Inport  Port=2
  rot3 : Inport  Port=3
  2 : Product
  3 : Product  Inputs=3
  7 : Product
  8 : Product  Inputs=3
  Combine : Concatenate  NumInputs=3  Mode=Multidimensional array  ConcatenateDimension=2
  Trigonometric Function{,1..2,6,9,11} (6 alike) : Trigonometry  Operator=cos
  Trigonometric Function{3..5,7..8,10} (6 alike) : Trigonometry
  rot11 : Product
  rot12 : Sum
  rot13 : Sum  Inputs=+-
  rot[1,1-3] : Outport
  wires:
  rot13/1 -> Combine/3
  8/1 -> rot13/2
  7/1 -> rot13/1
  Trigonometric Function11/1 -> 8/3
  Trigonometric Function10/1 -> 8/2
  Trigonometric Function9/1 -> 8/1
  Trigonometric Function8/1 -> 7/2
  Trigonometric Function7/1 -> 7/1
  rot1/1 -> Trigonometric Function7/1, Trigonometric Function9/1, Trigonometric Function4/1, Trigonometric Function2/1
  rot3/1 -> Trigonometric Function8/1, Trigonometric Function11/1, Trigonometric Function6/1, Trigonometric Function3/1, Trigonometric Function1/1
  rot2/1 -> Trigonometric Function10/1, Trigonometric Function5/1, Trigonometric Function/1
  Combine/1 -> rot[1,1-3]/1
  rot12/1 -> Combine/2
  3/1 -> rot12/2
  2/1 -> rot12/1
  Trigonometric Function6/1 -> 3/3
  Trigonometric Function5/1 -> 3/2
  Trigonometric Function4/1 -> 3/1
  Trigonometric Function3/1 -> 2/2
  Trigonometric Function2/1 -> 2/1
  rot11/1 -> Combine/1
  Trigonometric Function1/1 -> rot11/2
  Trigonometric Function/1 -> rot11/1

== system MPS_device_passive/PTO P4F4/VisuP4F1/Hydrodynamic Body/Morrison Element and ViscousDampingForceCalculation/Morrison Element Variant Subsystem/Morrison Element On/No Wave Morison Force/MorrisonElements/Rotation2 ==
  rot1 : Inport
  rot2 : Inport  Port=2
  rot3 : Inport  Port=3
  2 : Product
  3 : Product  Inputs=3
  7 : Product
  8 : Product  Inputs=3
  Combine : Concatenate  NumInputs=3  Mode=Multidimensional array  ConcatenateDimension=2
  Gain : Gain  Gain=-1
  Trigonometric Function{,2..3,8..9} (5 alike) : Trigonometry  Operator=cos
  Trigonometric Function{1,4..7,10..11} (7 alike) : Trigonometry
  rot11 : Product
  rot12 : Sum  Inputs=+-
  rot13 : Sum
  rot[2,1-3] : Outport
  wires:
  Gain/1 -> rot11/1
  rot13/1 -> Combine/3
  8/1 -> rot13/2
  7/1 -> rot13/1
  Trigonometric Function11/1 -> 8/3
  Trigonometric Function10/1 -> 8/2
  Trigonometric Function9/1 -> 8/1
  Trigonometric Function8/1 -> 7/2
  Trigonometric Function7/1 -> 7/1
  rot1/1 -> Trigonometric Function7/1, Trigonometric Function9/1, Trigonometric Function4/1, Trigonometric Function2/1
  rot3/1 -> Trigonometric Function8/1, Trigonometric Function11/1, Trigonometric Function6/1, Trigonometric Function3/1, Trigonometric Function1/1
  rot2/1 -> Trigonometric Function10/1, Trigonometric Function5/1, Trigonometric Function/1
  Combine/1 -> rot[2,1-3]/1
  rot12/1 -> Combine/2
  3/1 -> rot12/2
  2/1 -> rot12/1
  Trigonometric Function6/1 -> 3/3
  Trigonometric Function5/1 -> 3/2
  Trigonometric Function4/1 -> 3/1
  Trigonometric Function3/1 -> 2/2
  Trigonometric Function2/1 -> 2/1
  rot11/1 -> Combine/1
  Trigonometric Function1/1 -> rot11/2
  Trigonometric Function/1 -> Gain/1

== system MPS_device_passive/PTO P4F4/VisuP4F1/Hydrodynamic Body/Morrison Element and ViscousDampingForceCalculation/Morrison Element Variant Subsystem/Morrison Element On/No Wave Morison Force/MorrisonElements/Rotation3 ==
  rot1 : Inport
  rot2 : Inport  Port=2
  2 : Product
  7 : Product
  Combine : Concatenate  NumInputs=3  Mode=Multidimensional array  ConcatenateDimension=2
  Gain1 : Gain  Gain=-1
  TrigFun1 : Trigonometry
  TrigFun2 : Trigonometry
  TrigFun3 : Trigonometry  Operator=cos
  TrigFun4 : Trigonometry  Operator=cos
  TrigFun5 : Trigonometry  Operator=cos
  rot[3,1-3] : Outport
  wires:
  Gain1/1 -> 2/1
  TrigFun2/1 -> Gain1/1
  7/1 -> Combine/3
  rot1/1 -> TrigFun4/1, TrigFun2/1
  TrigFun5/1 -> 7/2
  TrigFun4/1 -> 7/1
  rot2/1 -> TrigFun1/1, TrigFun3/1, TrigFun5/1
  Combine/1 -> rot[3,1-3]/1
  2/1 -> Combine/2
  TrigFun3/1 -> 2/2
  TrigFun1/1 -> Combine/1

== system MPS_device_passive/PTO P4F4/VisuP4F1/Hydrodynamic Body/Morrison Element and ViscousDampingForceCalculation/Morrison Element Variant Subsystem/Morrison Element On/Regular Wave Morison Force/MorrisonElements/OrbitalVelocity ==
  Disp : Inport
  Time : Inport  Port=2
  MATLAB Function : MATLAB Function  TreatAsAtomicUnit=on
  WaveAmp : Constant  Value=waves.A(1,:)
  WaveFreq : Constant  Value=waves.w(1,:)
  WaveNumber : Constant  Value=waves.k(1,:)
  gravity : Constant  Value=simu.g  VectorParams1D=off
  phase : Constant  Value=0
  rampTime : Constant  Value=simu.rampT  VectorParams1D=off
  waterDepth : Constant  Value=waves.waterDepth  VectorParams1D=off
  waveDirection : Constant  Value=waves.waveDir  VectorParams1D=off
  u-V : Outport
  w-V : Outport  Port=2
  u-A : Outport  Port=3
  w-A : Outport  Port=4
  v-V : Outport  Port=5
  v-A : Outport  Port=6
  wires:
  MATLAB Function/5(ya) -> v-A/1
  MATLAB Function/1(u) -> u-V/1
  MATLAB Function/2(v) -> v-V/1
  MATLAB Function/6(za) -> w-A/1
  MATLAB Function/4(xa) -> u-A/1
  MATLAB Function/3(w) -> w-V/1
  rampTime/1 -> MATLAB Function/7(rampT)
  waveDirection/1 -> MATLAB Function/8(waveDir)
  waterDepth/1 -> MATLAB Function/9(waterDepth)
  gravity/1 -> MATLAB Function/10(g)
  Time/1 -> MATLAB Function/6(time)
  WaveAmp/1 -> MATLAB Function/4(waveAmp)
  WaveFreq/1 -> MATLAB Function/3(waveFreq)
  WaveNumber/1 -> MATLAB Function/2(waveNumber)
  phase/1 -> MATLAB Function/5(randPhase)
  Disp/1 -> MATLAB Function/1(disp)

== system MPS_device_passive/PTO P4F4/VisuP4F1/Hydrodynamic Body/Morrison Element and ViscousDampingForceCalculation/Morrison Element Variant Subsystem/Morrison Element On/Regular Wave Morison Force/MorrisonElements/Rotation1 ==
  rot1 : Inport
  rot2 : Inport  Port=2
  rot3 : Inport  Port=3
  2 : Product
  3 : Product  Inputs=3
  7 : Product
  8 : Product  Inputs=3
  Combine : Concatenate  NumInputs=3  Mode=Multidimensional array  ConcatenateDimension=2
  Trigonometric Function{,1..2,6,9,11} (6 alike) : Trigonometry  Operator=cos
  Trigonometric Function{3..5,7..8,10} (6 alike) : Trigonometry
  rot11 : Product
  rot12 : Sum
  rot13 : Sum  Inputs=+-
  rot[1,1-3] : Outport
  wires:
  rot13/1 -> Combine/3
  8/1 -> rot13/2
  7/1 -> rot13/1
  Trigonometric Function11/1 -> 8/3
  Trigonometric Function10/1 -> 8/2
  Trigonometric Function9/1 -> 8/1
  Trigonometric Function8/1 -> 7/2
  Trigonometric Function7/1 -> 7/1
  rot1/1 -> Trigonometric Function7/1, Trigonometric Function9/1, Trigonometric Function4/1, Trigonometric Function2/1
  rot3/1 -> Trigonometric Function8/1, Trigonometric Function11/1, Trigonometric Function6/1, Trigonometric Function3/1, Trigonometric Function1/1
  rot2/1 -> Trigonometric Function10/1, Trigonometric Function5/1, Trigonometric Function/1
  Combine/1 -> rot[1,1-3]/1
  rot12/1 -> Combine/2
  3/1 -> rot12/2
  2/1 -> rot12/1
  Trigonometric Function6/1 -> 3/3
  Trigonometric Function5/1 -> 3/2
  Trigonometric Function4/1 -> 3/1
  Trigonometric Function3/1 -> 2/2
  Trigonometric Function2/1 -> 2/1
  rot11/1 -> Combine/1
  Trigonometric Function1/1 -> rot11/2
  Trigonometric Function/1 -> rot11/1
